simulink model "HW1_1"  (R2025b)
settings: Solver=VariableStepAuto  StartTime=0.0  StopTime=20  RelTol=1e-3
libraries: simulink x1
settings Model: Creator=yunzhuorui  LastModifiedBy=yunzhuorui

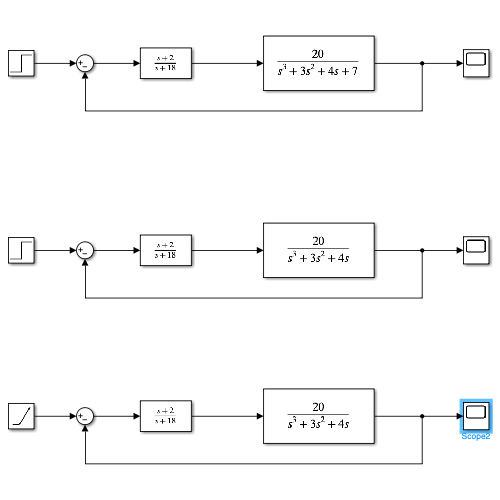
[thumbnail: Simulink's stored preview of the top-level diagram]
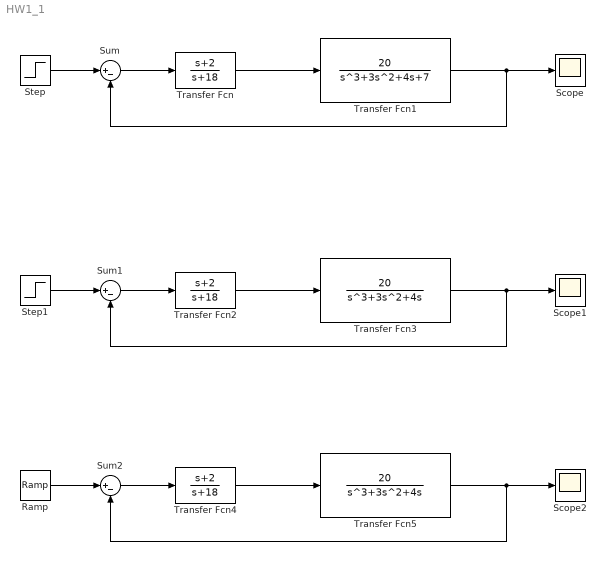
== system HW1_1 ==
  Ramp : simulink/Sources/Ramp  slope=5  start=0  InitialOutput=0
  Scope : Scope
      settings: ActiveDisplayYMinimum=-0.26089136088196324  ActiveDisplayYMaximum=2.34802224793767
  Scope1 : Scope
      settings: ActiveDisplayYMinimum=-0.624997829040837  ActiveDisplayYMaximum=5.6249804613675343
  Scope2 : Scope
      settings: ActiveDisplayYMinimum=-11.37500345023601  ActiveDisplayYMaximum=102.3750310521241  DataLoggingVariableName=ScopeData2
  Step : Step  After=5  SampleTime=0
  Step1 : Step  Time=0  After=5  SampleTime=0
  Sum : Sum  Inputs=|+-
  Sum1 : Sum  Inputs=|+-
  Sum2 : Sum  Inputs=|+-
  Transfer Fcn : TransferFcn  Numerator=[1 2]  Denominator=[1 18]
  Transfer Fcn1 : TransferFcn  Numerator=[20]  Denominator=[1 3 4 7]
  Transfer Fcn2 : TransferFcn  Numerator=[1 2]  Denominator=[1 18]
  Transfer Fcn3 : TransferFcn  Numerator=[20]  Denominator=[1 3 4 0]
  Transfer Fcn4 : TransferFcn  Numerator=[1 2]  Denominator=[1 18]
  Transfer Fcn5 : TransferFcn  Numerator=[20]  Denominator=[1 3 4 0]
  wires:
  Transfer Fcn/1 -> Transfer Fcn1/1
  Transfer Fcn1/1 -> Sum/2, Scope/1
  Step/1 -> Sum/1
  Sum/1 -> Transfer Fcn/1
  Step1/1 -> Sum1/1
  Sum1/1 -> Transfer Fcn2/1
  Transfer Fcn2/1 -> Transfer Fcn3/1
  Transfer Fcn3/1 -> Sum1/2, Scope1/1
  Ramp/1 -> Sum2/1
  Transfer Fcn4/1 -> Transfer Fcn5/1
  Sum2/1 -> Transfer Fcn4/1
  Transfer Fcn5/1 -> Sum2/2, Scope2/1
